simulink model "sensor_simulation"  (R2018a)
settings: Solver=VariableStepAuto  StartTime=0.0  StopTime=10.0  RelTol=1e-3
libraries: simulink x16
(part 2 of 2)

== system sensor_simulation/STATE ESTIMATION/ROLL EKF/CORRECTION STEP ==
  PREDICTED STATE : Inport
  PREDICTED COVARIANCE : Inport  Port=2
  MEASURED ROLL : Inport  Port=3
  MEASUREMENT COVARIANCE : Inport  Port=4
  EKF MEASUREMENT UPDATE : MATLAB Function  TreatAsAtomicUnit=on
  UPDATED STATE : Outport
  UPDATED COVARIANCE : Outport  Port=2
  wires:
  PREDICTED STATE/1 -> EKF MEASUREMENT UPDATE/1(predicted_state)
  PREDICTED COVARIANCE/1 -> EKF MEASUREMENT UPDATE/2(predicted_covariance)
  MEASURED ROLL/1 -> EKF MEASUREMENT UPDATE/3(measured_values)
  MEASUREMENT COVARIANCE/1 -> EKF MEASUREMENT UPDATE/4(R)
  EKF MEASUREMENT UPDATE/1(updated_state) -> UPDATED STATE/1
  EKF MEASUREMENT UPDATE/2(updated_covariance) -> UPDATED COVARIANCE/1

== system sensor_simulation/STATE ESTIMATION/ROLL EKF/PREDICTION STEP ==
  PREVIOUS STATE : Inport
  PREVIOUS COVARIANCE : Inport  Port=2
  A : Gain
  ADD Q : Sum
  AT : Gain
  PROCESS NOISE : Constant  Value=0.001
  STATE TRANSITION : Gain
  PREDICTED STATE : Outport
  PREDICTED COVARIANCE : Outport  Port=2
  wires:
  PREVIOUS STATE/1 -> STATE TRANSITION/1
  STATE TRANSITION/1 -> PREDICTED STATE/1
  PREVIOUS COVARIANCE/1 -> A/1
  A/1 -> AT/1
  AT/1 -> ADD Q/1
  PROCESS NOISE/1 -> ADD Q/2
  ADD Q/1 -> PREDICTED COVARIANCE/1

== system sensor_simulation/STATE ESTIMATION/YAW EKF/CORRECTION STEP ==
  PREDICTED STATE : Inport
  PREDICTED COVARIANCE : Inport  Port=2
  MEASURED YAW : Inport  Port=3
  MEASUREMENT COVARIANCE : Inport  Port=4
  EKF MEASUREMENT UPDATE : MATLAB Function  TreatAsAtomicUnit=on
  UPDATED STATE : Outport
  UPDATED COVARIANCE : Outport  Port=2
  wires:
  PREDICTED STATE/1 -> EKF MEASUREMENT UPDATE/1(predicted_state)
  PREDICTED COVARIANCE/1 -> EKF MEASUREMENT UPDATE/2(predicted_covariance)
  MEASURED YAW/1 -> EKF MEASUREMENT UPDATE/3(measured_values)
  MEASUREMENT COVARIANCE/1 -> EKF MEASUREMENT UPDATE/4(R)
  EKF MEASUREMENT UPDATE/1(updated_state) -> UPDATED STATE/1
  EKF MEASUREMENT UPDATE/2(updated_covariance) -> UPDATED COVARIANCE/1

== system sensor_simulation/STATE ESTIMATION/YAW EKF/PREDICTION STEP ==
  PREVIOUS STATE : Inport
  PREVIOUS COVARIANCE : Inport  Port=2
  A : Gain
  ADD Q : Sum
  AT : Gain
  PROCESS NOISE : Constant  Value=0.001
  STATE TRANSITION : Gain
  PREDICTED STATE : Outport
  PREDICTED COVARIANCE : Outport  Port=2
  wires:
  PREVIOUS STATE/1 -> STATE TRANSITION/1
  STATE TRANSITION/1 -> PREDICTED STATE/1
  PREVIOUS COVARIANCE/1 -> A/1
  A/1 -> AT/1
  AT/1 -> ADD Q/1
  PROCESS NOISE/1 -> ADD Q/2
  ADD Q/1 -> PREDICTED COVARIANCE/1

== matlab function sensor_simulation/STATE ESTIMATION/ROLL EKF/CORRECTION STEP/EKF MEASUREMENT UPDATE ==
  data: predicted_state input; updated_state output; predicted_covariance input; measured_values input; R input; updated_covariance output
function [updated_state,updated_covariance] = ...
KF_Update(predicted_state,predicted_covariance,measured_values,R)

innovation = measured_values - predicted_state;

S = predicted_covariance + R;

K = predicted_covariance / S;

updated_state = predicted_state + K*innovation;

updated_covariance = (1-K)*predicted_covariance;

== matlab function sensor_simulation/STATE ESTIMATION/PITCH EKF/CORRECTION STEP/EKF MEASUREMENT UPDATE ==
  data: predicted_state input; updated_state output; predicted_covariance input; measured_pitch input; R input; updated_covariance output
function [updated_state,updated_covariance] = ...
KF_Update(predicted_state,predicted_covariance,measured_pitch,R)

innovation = measured_pitch - predicted_state;

S = predicted_covariance + R;

K = predicted_covariance / S;

updated_state = predicted_state + K*innovation;

updated_covariance = (1-K)*predicted_covariance;

== matlab function sensor_simulation/STATE ESTIMATION/YAW EKF/CORRECTION STEP/EKF MEASUREMENT UPDATE ==
  data: predicted_state input; updated_state output; predicted_covariance input; measured_values input; R input; updated_covariance output
function [updated_state,updated_covariance] = ...
KF_Update(predicted_state,predicted_covariance,measured_values,R)

innovation = measured_values - predicted_state;

S = predicted_covariance + R;

K = predicted_covariance / S;

updated_state = predicted_state + K*innovation;

updated_covariance = (1-K)*predicted_covariance;

== matlab function sensor_simulation/STATE ESTIMATION/ALTITUDE EKF/CORRECTION STEP/EKF MEASUREMENT UPDATE ==
  data: predicted_state input; updated_state output; predicted_covariance input; measured_values input; R input; updated_covariance output
function [updated_state,updated_covariance] = ...
KF_Update(predicted_state,predicted_covariance,measured_values,R)

innovation = measured_values - predicted_state;

S = predicted_covariance + R;

K = predicted_covariance / S;

updated_state = predicted_state + K*innovation;

updated_covariance = (1-K)*predicted_covariance;

== matlab function sensor_simulation/STATE ESTIMATION/AIRSPEED EKF/CORRECTION STEP/EKF MEASUREMENT UPDATE ==
  data: predicted_state input; updated_state output; predicted_covariance input; measured_values input; R input; updated_covariance output
function [updated_state,updated_covariance] = ...
KF_Update(predicted_state,predicted_covariance,measured_values,R)

innovation = measured_values - predicted_state;

S = predicted_covariance + R;

K = predicted_covariance / S;

updated_state = predicted_state + K*innovation;

updated_covariance = (1-K)*predicted_covariance;
